simulink model "lin_3d"  (R2020b)
settings: Solver=ode1  StartTime=0.0  StopTime=600  FixedStep=0.001  RelTol=1e-3  EnableMultiTasking=on
values from neighbouring files (symbols this model uses):
  beta3d = 0.9    [simulate_hover.m]
  cycleGain = 0.5    [advanced_model_setup.m]    (also in setup_physical.m = 1; simulate_hover.m = 0.2)
  epsilon3d = evalin('base', 'epsilon3d')    [gainScheduling.m]    (also in simulate_hover.m = 1)
  K = lqi(sys, Q, R)    [gainScheduling.m]    (also in setup_lab_hover.m = K1; simulate_hover.m)
  k3d = evalin('base', 'k3d')    [gainScheduling.m]    (also in simulate_hover.m = 1.65)
  K_AMP = 3    [advanced_model_setup.m]    (also in setup_lab_hover.m; setup_physical.m; simulate_hover.m)
  K_EC_P = 2 * pi / ( 8 * 1024 )    (= 0.000766990393943)    [advanced_model_setup.m]    (also in setup_lab_hover.m; setup_physical.m; simulate_hover.m)
  K_EC_R = 2 * pi / ( 8 * 1024 )    (= 0.000766990393943)    [advanced_model_setup.m]    (also in setup_lab_hover.m; setup_physical.m; simulate_hover.m)
  K_EC_Y = -2 * pi / ( 8 * 1024 )    (= -0.000766990393943)    [advanced_model_setup.m]    (also in setup_lab_hover.m; setup_physical.m; simulate_hover.m)
  u00_range = [-11 -10.5 -10 -9.5 -9 -8.5 -8 -7.5 -7 -6.5 -6 -5.5 ... (45 elements, 1x45)]    [lookup_lin3d.mat]    (also in lookup_nonlin3d.mat; lookup_nonlin_pitchyaw.mat = [-11 -10.9 -10.8 -10.7 -10.6 -10.5 -10.4 -10.3 -10.2 -10.1 -)
  u10_range = -40:0.00001:40    [lookup_gen_5.m]    (also in lookup_gen_optimal.m = -3:0.2:3; lookup_lin3d.mat = [-11 -10.5 -10 -9.5 -9 -8.5 -8 -7.5 -7 -6.5 -6 -5.5 ... (45 ; lookup_nonlin3d.mat = [-11 -10.5 -10 -9.5 -9 -8.5 -8 -7.5 -7 -6.5 -6 -5.5 ... (45 ; lookup_nonlin_pitchyaw.mat = [-11 -10.9 -10.8 -10.7 -10.6 -10.5 -10.4 -10.3 -10.2 -10.1 -)
  u1_T = zeros(x5L, x6L, u10L, u20L)    [lookup_gen_optimal.m]    (also in lookup_lin3d.mat = [-8.91749108301 -9.05775625381 -9.19802070914 -9.33828594207; lookup_nonlin3d.mat = [-10.7844387629 -10.8648620301 -10.9452851893 -11.0257085566; lookup_nonlin_pitchyaw.mat = [-10.9045735396 -10.9207431106 -10.936911981 -10.953081676 -)
  u20_range = -40:0.00001:40    [lookup_gen_5.m]    (also in lookup_gen_optimal.m = -3:0.2:3; lookup_lin3d.mat = [-11 -10.5 -10 -9.5 -9 -8.5 -8 -7.5 -7 -6.5 -6 -5.5 ... (45 ; lookup_nonlin3d.mat = [-11 -10.5 -10 -9.5 -9 -8.5 -8 -7.5 -7 -6.5 -6 -5.5 ... (45 ; lookup_nonlin_pitchyaw.mat = [-11 -10.5 -10 -9.5 -9 -8.5 -8 -7.5 -7 -6.5 -6 -5.5 ... (45 )
  u2_T = zeros(x5L, x6L, u10L, u20L)    [lookup_gen_optimal.m]    (also in lookup_lin3d.mat = [11.9999976349 11.9999976348 11.9999995269 11.9999995269 11.; lookup_nonlin3d.mat = [11.999999986 11.9999999853 11.9999999846 11.9999999837 11.9; lookup_nonlin_pitchyaw.mat = [11.9999999849 11.9999999848 11.9999996928 11.9999999845 11.)
  u3_T = zeros(x5L, x6L, u10L, u20L)    [lookup_gen_optimal.m]    (also in lookup_lin3d.mat = [-11.9999984131 -11.9999984131 -11.9999996826 -11.9999996826; lookup_nonlin3d.mat = [-11.999999986 -11.9999999853 -11.9999999846 -11.9999999837 ; lookup_nonlin_pitchyaw.mat = [-11.9999999699 -11.9999999696 -11.9999993856 -11.999999969 )
  u4_T = zeros(x5L, x6L, u10L, u20L)    [lookup_gen_optimal.m]    (also in lookup_lin3d.mat = [11.9999951772 11.9999951773 11.9999990355 11.9999990356 11.; lookup_nonlin3d.mat = [10.7844387816 10.8648620565 10.9452851985 11.0257085566 11.; lookup_nonlin_pitchyaw.mat = [-11.9999999699 -11.9999999696 -11.9999993856 -11.999999969 )
  V_bias = 12    [advanced_model_setup.m]    (also in setup_lab_hover.m; setup_physical.m; simulate_hover.m)
  VMAX_AMP = 24    [advanced_model_setup.m]    (also in setup_lab_hover.m; setup_physical.m; simulate_hover.m)
  wcf = 2 * pi * 20    (= 125.663706144)    [advanced_model_setup.m]    (also in setup_lab_hover.m; setup_physical.m; simulate_hover.m = 628.318530718)
  x1_traj = x1_traj*pi/180    [lookup_approxLimit.m]    (also in lookup_approxLimit3d.m)
  x1_trajectory = zeros(x1TL, x2TL)    [lookup_approxLimit.m]    (also in lookup_approxLimit3d.m = zeros(x1TL, x2TL, x3TL))
  x2_traj = x2_traj*pi/180    [lookup_approxLimit.m]    (also in lookup_approxLimit3d.m)
  x2_trajectory = zeros(x1TL, x2TL)    [lookup_approxLimit.m]    (also in lookup_approxLimit3d.m = zeros(x1TL, x2TL, x3TL))
  x3_traj = x3_traj*pi/180    [lookup_approxLimit3d.m]
  x3_trajectory = zeros(x1TL, x2TL, x3TL)    [lookup_approxLimit3d.m]
  zetaf = 0.6    [advanced_model_setup.m]    (also in setup_lab_hover.m; setup_physical.m; simulate_hover.m)
undefined symbols (not defined in the file or in its folder): HIL, qc_get_step_size
libraries: simulink_extras x5, quarc_library x3
settings Model: SimulationMode=external  ExtModeTrigDuration=10000  Creator=hpineros  LastModifiedBy=256444
settings SolverCC: PositivePriorityOrder=on
settings DataIOCC: MaxDataPoints=5000  SaveFormat=Array  SignalLoggingSaveFormat=ModelDataLogs  InspectSignalLogs=on  ReturnWorkspaceOutputs=off
settings OptimizationCC: ExpressionDepthLimit=2147483647  InitFltsAndDblsToZero=on  LifeSpan=inf
settings DebuggingCC: SaveWithParameterizedLinksMsg=none  UnderspecifiedInitializationDetection=Classic  MergeDetectMultiDrivingBlocksExec=none  SolverPrmCheckMsg=warning  FcnCallInpInsideContextMsg=warning  StateNameClashWarn=warning  SFUnexpectedBacktrackingDiag=warning  SFNoUnconditionalDefaultTransitionDiag=warning  SFExecutionAtInitializationDiag=none  ArithmeticOperatorsInVariantConditions=warning
settings HardwareCC: ProdBitPerPointer=32  ProdBitPerSizeT=32  ProdBitPerPtrDiffT=32  ProdLargestAtomicFloat=None  ProdIntDivRoundTo=Undefined  ProdEndianess=Unspecified  ProdWordSize=32  ProdHWDeviceType=32-bit Generic
settings ModelReferenceCC: PropagateSignalLabelsOutOfModel=off
settings SFSimCC: SimUseLocalCustomCode=off  CustomCodeUndefinedFunction=UseInterfaceOnly
settings RTWCC: Description=QUARC Win64 Target  SystemTargetFile=quarc_win64.tlc  TemplateMakefile=quarc_default_tmf  RTWUseLocalCustomCode=off
settings CodeAppCC: StateflowObjectComments=on
settings STFCustomTargetCC: CombineOutputUpdateFcns=on  GRTInterface=off
settings GRTTargetCC: TargetLangStandard=C89/C90 (ANSI)  ParMdlRefBuildCompliant=off  CompOptLevelCompliant=off  MatFileLogging=off  UseToolchainInfoCompliant=off  ExtMode=on  ExtModeMexFile=quarc_comm
settings ConfigComp: CovMetricSettings=dw  CovSaveCumulativeToWorkspaceVar=on  CovSaveSingleToWorkspaceVar=on  CovExternalEMLEnable=off

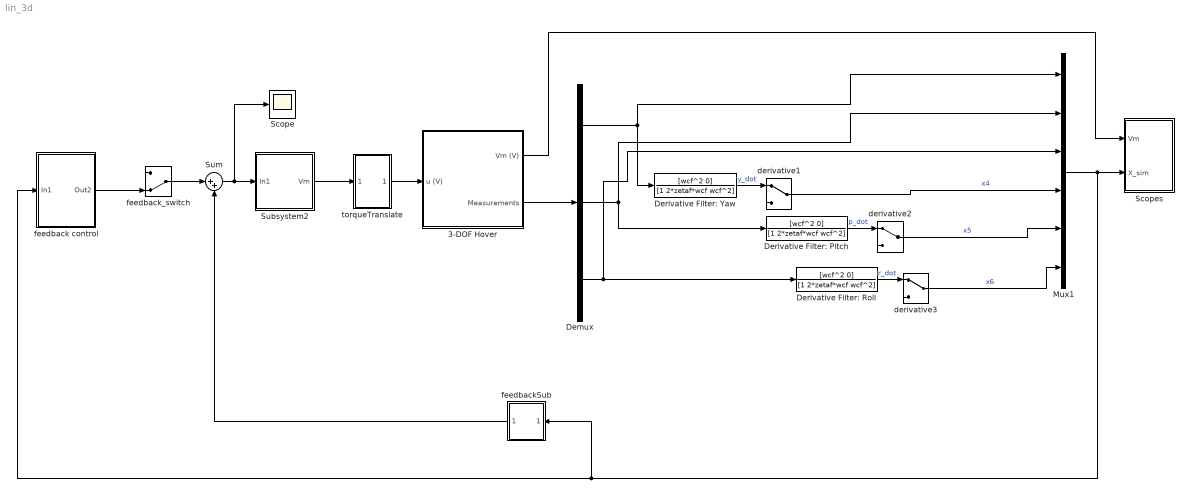
== system lin_3d ==
  3-DOF Hover : Subsystem
  Demux : Demux  Outputs=3
  Derivative Filter: Pitch : TransferFcn  Numerator=[wcf^2 0]  Denominator=[1 2*zetaf*wcf wcf^2]
  Derivative Filter: Roll : TransferFcn  Numerator=[wcf^2 0]  Denominator=[1 2*zetaf*wcf wcf^2]
  Derivative Filter: Yaw : TransferFcn  Numerator=[wcf^2 0]  Denominator=[1 2*zetaf*wcf wcf^2]
  Mux1 : Mux  Inputs=6
  Scope : Scope
  Scopes : Subsystem
  Subsystem2 : Subsystem
  Sum : Sum  Inputs=|++
  derivative1 : ManualSwitch
  derivative2 : ManualSwitch
  derivative3 : ManualSwitch
  feedback control : Subsystem
  feedbackSub : Subsystem
  feedback_switch : ManualSwitch  CurrentSetting=0
  torqueTranslate : Subsystem
  wires:
  Demux/3 -> Mux1/3, Derivative Filter: Roll/1
  Demux/1 -> Mux1/1, Derivative Filter: Yaw/1
  derivative2/1 -> Mux1/5  "x5"
  derivative1/1 -> Mux1/4  "x4"
  Demux/2 -> Mux1/2, Derivative Filter: Pitch/1
  Derivative Filter: Pitch/1 -> derivative2/1  "p_dot"
  Derivative Filter: Roll/1 -> derivative3/1  "r_dot"
  Derivative Filter: Yaw/1 -> derivative1/1  "y_dot"
  3-DOF Hover/2(Measurements) -> Demux/1
  derivative3/1 -> Mux1/6  "x6"
  3-DOF Hover/1(Vm (V)) -> Scopes/1(Vm)
  Mux1/1 -> feedbackSub/1(Input), feedback control/1(In1), Scopes/2(X_sim)
  torqueTranslate/1(Out1) -> 3-DOF Hover/1(u (V))
  feedback_switch/1 -> Sum/1
  feedback control/1(Out2) -> feedback_switch/2
  Sum/1 -> Scope/1, Subsystem2/1(In1)
  Subsystem2/1(Vm) -> torqueTranslate/1(Vm)
  feedbackSub/1(Out1) -> Sum/2

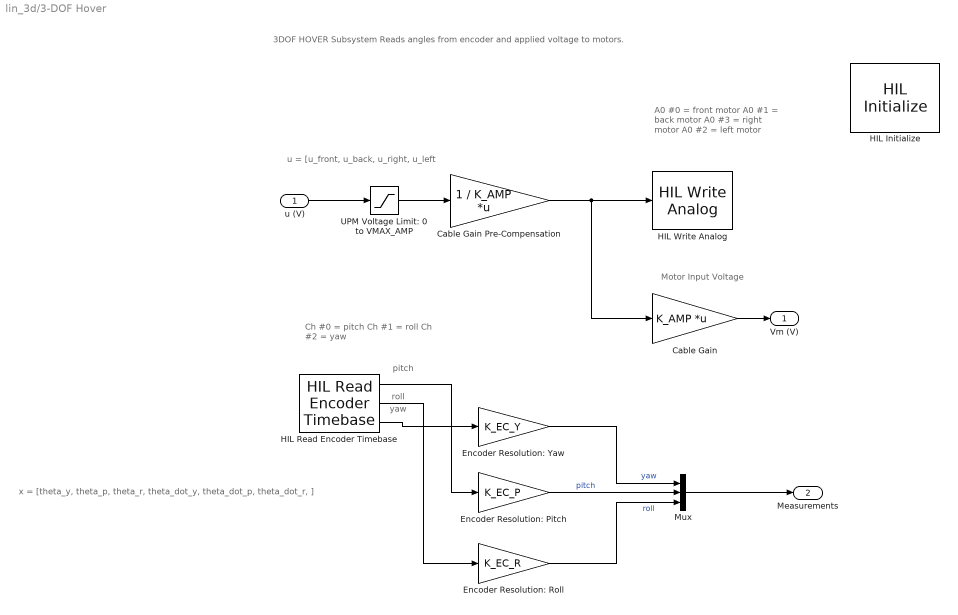
== system lin_3d/3-DOF Hover ==
  note: roll
  note: pitch
  note: yaw
  note: Motor Input Voltage
  note: x = [theta_y, theta_p, theta_r, theta_dot_y, theta_dot_p, theta_dot_r, ]
  note: A0 #0 = front motor
      | A0 #1 = back motor
      | A0 #3 = right motor
      | A0 #2 = left motor
  note: u = [u_front, u_back, u_right, u_left
  note: 3DOF HOVER Subsystem
      | Reads angles from encoder and applied voltage to motors.
  note: Ch #0 = pitch
      | Ch #1 = roll
      | Ch #2 = yaw
  u (V) : Inport
  Cable Gain : Gain  Gain=K_AMP  Multiplication=Matrix(K*u)  SaturateOnIntegerOverflow=on  OutDataTypeStr=Inherit: Same as input  ParamDataTypeStr=Inherit: Same as input
  Cable Gain Pre-Compensation : Gain  Gain=1 / K_AMP  Multiplication=Matrix(K*u)  SaturateOnIntegerOverflow=on  OutDataTypeStr=Inherit: Same as input  ParamDataTypeStr=Inherit: Same as input
  Encoder Resolution: Pitch : Gain  Gain=K_EC_P
  "Encoder Resolution: Roll " : Gain  Gain=K_EC_R
  Encoder Resolution: Yaw : Gain  Gain=K_EC_Y
  HIL Initialize : quarc_library/Data Acquisition/Generic/Configuration/HIL Initialize  object_name=HIL-1  board_type=q8_usb  board_number=0  board_options=update_rate=normal  exclusive=off  active=on  hardware_clocks=[0:2]  clock_modes=[]  initial_clock_frequencies=[]  set_clock_params_at_start=off  set_clock_params_at_switch_in=off  set_clock_frequencies_at_start=off  set_clock_frequencies_at_switch_in=off  analog_input_channels=[0:7]  analog_input_configurations=[]  analog_input_maximums=10  analog_input_minimums=-10  set_analog_input_params_at_start=on  set_analog_input_params_at_switch_in=off  analog_output_channels=[0:7]  analog_output_maximums=10  analog_output_minimums=-10  initial_analog_outputs=[0]  final_analog_outputs=[0]  watchdog_analog_outputs=0  set_analog_output_params_at_start=on  set_analog_output_params_at_switch_in=off  set_analog_outputs_at_start=on  set_analog_outputs_at_switch_in=off  set_analog_outputs_at_terminate=on  set_analog_outputs_at_switch_out=off  set_analog_outputs_on_watchdog=off  digital_input_channels=[]  digital_output_channels=[0:3]  digital_output_configuration=[]  initial_digital_outputs=[0]  final_digital_outputs=[0]  watchdog_digital_outputs=[0]  set_digital_output_params_at_start=off  set_digital_output_params_at_switch_in=off  set_digital_outputs_at_start=on  set_digital_outputs_at_switch_in=off  set_digital_outputs_at_terminate=on  set_digital_outputs_at_switch_out=off  set_digital_outputs_on_watchdog=off  encoder_channels=[0:7]  quadrature=[4]  encoder_filter_frequency=[]  initial_encoder_counts=[0]  set_encoder_params_at_start=on  set_encoder_params_at_switch_in=off  set_encoder_counts_at_start=on  set_encoder_counts_at_switch_in=off  pwm_channels=[0:7]  pwm_modes=0  pwm_frequency=99.532799999999995e6/4095  pwm_configuration=[0]  pwm_alignment=[0]  pwm_polarity=[1]  pwm_leading_deadband=[0]  pwm_trailing_deadband=[0]  initial_pwm_outputs=[0]  final_pwm_outputs=[0]  watchdog_pwm_outputs=[0]  set_pwm_params_at_start=on  set_pwm_params_at_switch_in=off  set_pwm_outputs_at_start=on  set_pwm_outputs_at_switch_in=off  set_pwm_outputs_at_terminate=on  set_pwm_outputs_at_switch_out=off  set_pwm_outputs_on_watchdog=off  other_output_channels=[]  initial_other_outputs=[]  final_other_outputs=[]  watchdog_other_outputs=[]  set_other_outputs_at_start=off  set_other_outputs_at_switch_in=off  set_other_outputs_at_terminate=off  set_other_outputs_at_switch_out=off  set_other_outputs_on_watchdog=off
  HIL Read Encoder Timebase : quarc_library/Data Acquisition/Generic/Timebases/HIL Read Encoder Timebase  object_name=HIL-1  clock=0  channels=[0:2]  active=on  vector_output=off  data_type_mode=Inherit via back propagation  data_type=double  overflow_mode=Error on overflow  samples_in_buffer=max(ceil(1/qc_get_step_size), 1)
  HIL Write Analog : quarc_library/Data Acquisition/Generic/Immediate I//O/HIL Write Analog  object_name=HIL-1  channels=[0,1,2,3]  sample_time=-1  active=off  vector_input=on
  Mux : Mux  Inputs=3
  UPM Voltage Limit: 0 to VMAX_AMP : Saturate  UpperLimit=VMAX_AMP  LowerLimit=0
  Vm (V) : Outport
  Measurements : Outport  Port=2
  wires:
  Cable Gain Pre-Compensation/1 -> Cable Gain/1, HIL Write Analog/1
  HIL Read Encoder Timebase/3 -> Encoder Resolution: Yaw/1
  HIL Read Encoder Timebase/1 -> Encoder Resolution: Pitch/1
  HIL Read Encoder Timebase/2 -> "Encoder Resolution: Roll "/1
  UPM Voltage Limit: 0 to VMAX_AMP/1 -> Cable Gain Pre-Compensation/1
  Cable Gain/1 -> Vm (V)/1
  u (V)/1 -> UPM Voltage Limit: 0 to VMAX_AMP/1
  "Encoder Resolution: Roll "/1 -> Mux/3  "roll"
  Encoder Resolution: Yaw/1 -> Mux/1  "yaw"
  Encoder Resolution: Pitch/1 -> Mux/2  "pitch"
  Mux/1 -> Measurements/1

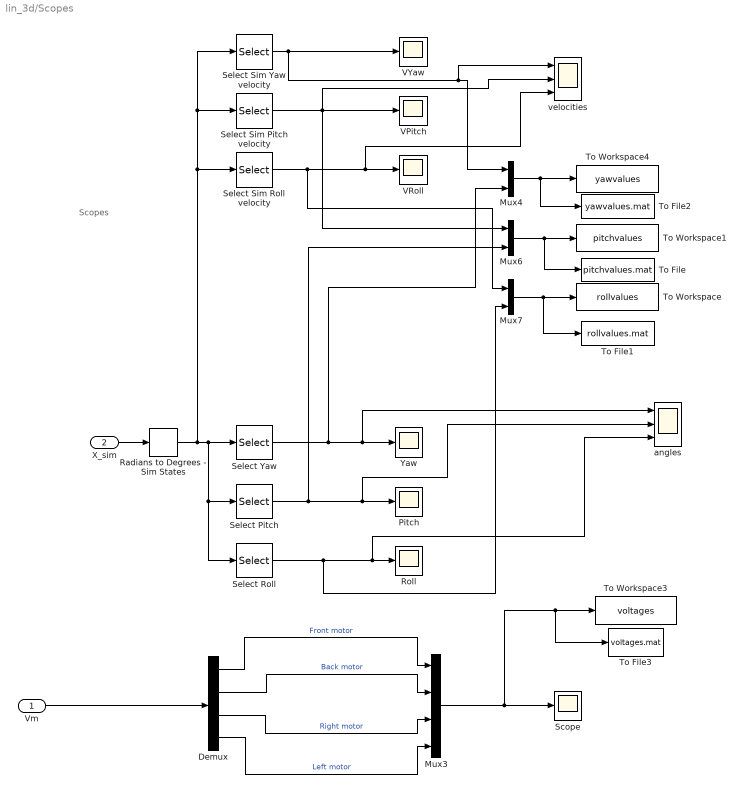
== system lin_3d/Scopes ==
  note: Scopes
  Vm : Inport
  X_sim : Inport  Port=2
  Demux : Demux
  Mux3 : Mux
  Mux4 : Mux  Inputs=2
  Mux6 : Mux  Inputs=2
  Mux7 : Mux  Inputs=2
  Pitch : Scope
  Radians to Degrees - Sim States : simulink_extras/Transformations/Radians to Degrees
  Roll : Scope
  Scope : Scope
  Select Pitch : Selector  InputPortWidth=6  IndexOptions=Index vector (dialog)  Indices=2  OutputSizes=1
  Select Roll : Selector  InputPortWidth=6  IndexOptions=Index vector (dialog)  Indices=3  OutputSizes=1
  Select Sim Pitch velocity : Selector  InputPortWidth=6  IndexOptions=Index vector (dialog)  Indices=5  OutputSizes=1
  Select Sim Roll velocity : Selector  InputPortWidth=6  IndexOptions=Index vector (dialog)  Indices=6  OutputSizes=1
  Select Sim Yaw velocity : Selector  InputPortWidth=6  IndexOptions=Index vector (dialog)  Indices=4  OutputSizes=1
  Select Yaw : Selector  InputPortWidth=6  IndexOptions=Index vector (dialog)  Indices=1  OutputSizes=1
  To File : ToFile  Filename=pitchvalues.mat
  To File1 : ToFile  Filename=rollvalues.mat
  To File2 : ToFile  Filename=yawvalues.mat
  To File3 : ToFile  Filename=voltages.mat
  To Workspace : ToWorkspace  VariableName=rollvalues  SampleTime=-1
  To Workspace1 : ToWorkspace  VariableName=pitchvalues  SampleTime=-1
  To Workspace3 : ToWorkspace  VariableName=voltages  SampleTime=-1
  To Workspace4 : ToWorkspace  VariableName=yawvalues  SampleTime=-1
  VPitch : Scope
  VRoll : Scope
  VYaw : Scope
  Yaw : Scope
  angles : Scope  NumInputPorts=3
  velocities : Scope  NumInputPorts=3
  wires:
  Select Roll/1 -> angles/3, Roll/1, Mux7/2
  Radians to Degrees - Sim States/1 -> Select Sim Roll velocity/1, Select Sim Pitch velocity/1, Select Sim Yaw velocity/1, Select Roll/1, Select Pitch/1, Select Yaw/1
  Select Pitch/1 -> angles/2, Pitch/1, Mux6/2
  X_sim/1 -> Radians to Degrees - Sim States/1
  Demux/1 -> Mux3/1  "Front motor"
  Demux/2 -> Mux3/2  "Back motor"
  Demux/3 -> Mux3/3  "Right motor"
  Demux/4 -> Mux3/4  "Left motor"
  Vm/1 -> Demux/1
  Select Sim Yaw velocity/1 -> VYaw/1, velocities/1, Mux4/1
  Select Sim Roll velocity/1 -> velocities/3, VRoll/1, Mux7/1
  Select Sim Pitch velocity/1 -> Mux6/1, velocities/2, VPitch/1
  Mux3/1 -> To File3/1, To Workspace3/1, Scope/1
  Select Yaw/1 -> angles/1, Yaw/1, Mux4/2
  Mux7/1 -> To File1/1, To Workspace/1
  Mux6/1 -> To File/1, To Workspace1/1
  Mux4/1 -> To File2/1, To Workspace4/1

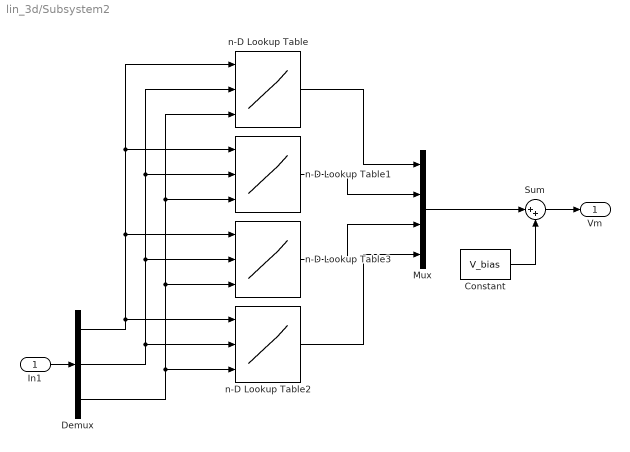
== system lin_3d/Subsystem2 ==
  In1 : Inport
  Constant : Constant  Value=V_bias
  Demux : Demux  Outputs=3
  Mux : Mux
  Sum : Sum  Inputs=|++
  n-D Lookup Table : Lookup_n-D  NumberOfTableDimensions=3  BreakpointsForDimension1=u00_range  BreakpointsForDimension2=u10_range  BreakpointsForDimension3=u20_range  BreakpointsForDimension4=u10_range  BreakpointsForDimension5=u20_range  Table=u1_T  InternalRulePriority=Speed  RndMeth=Simplest  InputSameDT=on
      settings: InputPortMap=u0,u1,u2
  n-D Lookup Table1 : Lookup_n-D  NumberOfTableDimensions=3  BreakpointsForDimension1=u00_range  BreakpointsForDimension2=u10_range  BreakpointsForDimension3=u20_range  BreakpointsForDimension4=u10_range  BreakpointsForDimension5=u20_range  Table=u2_T  InternalRulePriority=Speed  RndMeth=Simplest  InputSameDT=on
      settings: InputPortMap=u0,u1,u2
  n-D Lookup Table2 : Lookup_n-D  NumberOfTableDimensions=3  BreakpointsForDimension1=u00_range  BreakpointsForDimension2=u10_range  BreakpointsForDimension3=u20_range  BreakpointsForDimension4=u10_range  BreakpointsForDimension5=u20_range  Table=u4_T  InternalRulePriority=Speed  RndMeth=Simplest  InputSameDT=on
      settings: InputPortMap=u0,u1,u2
  n-D Lookup Table3 : Lookup_n-D  NumberOfTableDimensions=3  BreakpointsForDimension1=u00_range  BreakpointsForDimension2=u10_range  BreakpointsForDimension3=u20_range  BreakpointsForDimension4=u10_range  BreakpointsForDimension5=u20_range  Table=u3_T  InternalRulePriority=Speed  RndMeth=Simplest  InputSameDT=on
      settings: InputPortMap=u0,u1,u2
  Vm : Outport
  wires:
  Sum/1 -> Vm/1
  Mux/1 -> Sum/1
  Constant/1 -> Sum/2
  In1/1 -> Demux/1
  n-D Lookup Table/1 -> Mux/1
  n-D Lookup Table1/1 -> Mux/2
  n-D Lookup Table3/1 -> Mux/3
  n-D Lookup Table2/1 -> Mux/4
  Demux/1 -> n-D Lookup Table2/1, n-D Lookup Table3/1, n-D Lookup Table/1, n-D Lookup Table1/1
  Demux/3 -> n-D Lookup Table2/3, n-D Lookup Table3/3, n-D Lookup Table1/3, n-D Lookup Table/3
  Demux/2 -> n-D Lookup Table2/2, n-D Lookup Table3/2, n-D Lookup Table1/2, n-D Lookup Table/2

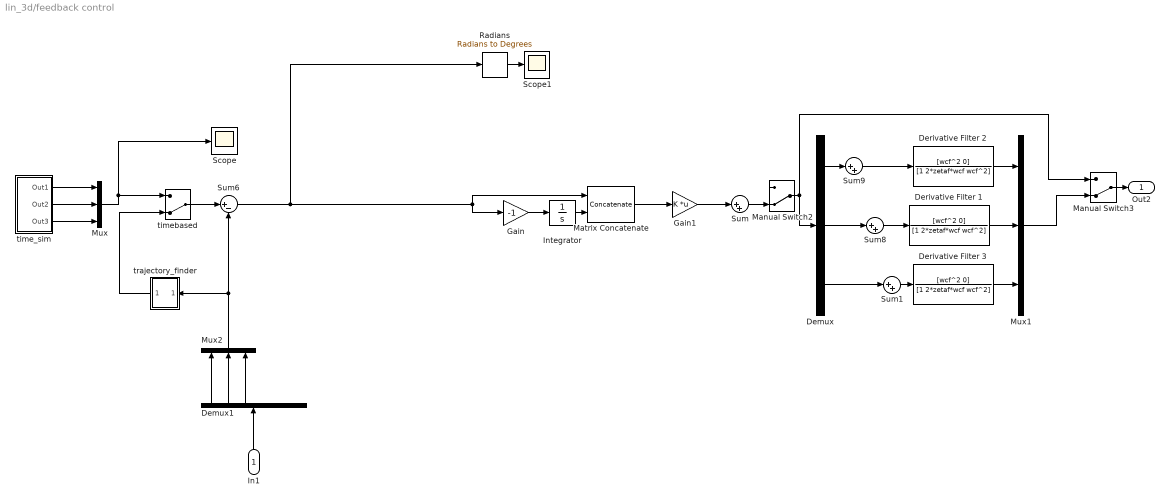
== system lin_3d/feedback control ==
  In1 : Inport
  Demux : Demux  Outputs=3
  Demux1 : Demux  Outputs=6
  Derivative Filter 1 : TransferFcn  Numerator=[wcf^2 0]  Denominator=[1 2*zetaf*wcf wcf^2]
  Derivative Filter 2 : TransferFcn  Numerator=[wcf^2 0]  Denominator=[1 2*zetaf*wcf wcf^2]
  Derivative Filter 3 : TransferFcn  Numerator=[wcf^2 0]  Denominator=[1 2*zetaf*wcf wcf^2]
  Gain : Gain  Gain=-1
  Gain1 : Gain  Gain=K  Multiplication=Matrix(K*u)
  Integrator : Integrator
  Manual Switch2 : ManualSwitch  CurrentSetting=0
  Manual Switch3 : ManualSwitch  CurrentSetting=0
  Matrix Concatenate : Concatenate  Mode=Multidimensional array
  Mux : Mux  Inputs=3
  Mux1 : Mux  Inputs=3
  Mux2 : Mux  Inputs=3
  Radians : simulink_extras/Transformations/Radians to Degrees
  Scope : Scope
  Scope1 : Scope
  Sum{,1,8..9} (4 alike) : Sum  Inputs=|++
  Sum6 : Sum  Inputs=|+-
  time_sim : Subsystem
  timebased : ManualSwitch  CurrentSetting=0
  trajectory_finder : Subsystem
  Out2 : Outport
  wires:
  Mux/1 -> timebased/1, Scope/1
  Demux1/2 -> Mux2/2
  Demux1/1 -> Mux2/1
  Demux1/3 -> Mux2/3
  In1/1 -> Demux1/1
  Mux2/1 -> Sum6/2, trajectory_finder/1(Input)
  time_sim/1(Out1) -> Mux/1
  time_sim/2(Out2) -> Mux/2
  time_sim/3(Out3) -> Mux/3
  Demux/1 -> Sum9/1
  Demux/2 -> Sum8/1
  Derivative Filter 1/1 -> Mux1/2
  Manual Switch3/1 -> Out2/1
  Radians/1 -> Scope1/1
  Sum/1 -> Manual Switch2/2
  Manual Switch2/1 -> Manual Switch3/1, Demux/1
  Derivative Filter 2/1 -> Mux1/1
  Sum8/1 -> Derivative Filter 1/1
  Mux1/1 -> Manual Switch3/2
  Sum9/1 -> Derivative Filter 2/1
  Sum1/1 -> Derivative Filter 3/1
  Derivative Filter 3/1 -> Mux1/3
  Demux/3 -> Sum1/1
  timebased/1 -> Sum6/1
  trajectory_finder/1(Output) -> timebased/2
  Sum6/1 -> Radians/1, Matrix Concatenate/1, Gain/1
  Gain/1 -> Integrator/1
  Integrator/1 -> Matrix Concatenate/2
  Gain1/1 -> Sum/1
  Matrix Concatenate/1 -> Gain1/1

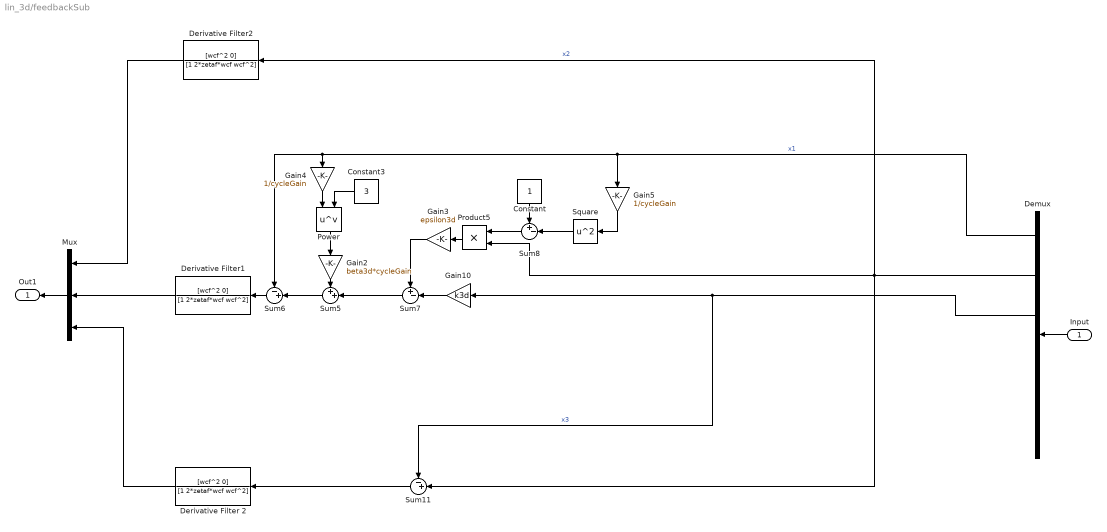
== system lin_3d/feedbackSub ==
  Input : Inport
  Constant : Constant
  Constant3 : Constant  Value=3
  Demux : Demux  Outputs=6
  Derivative Filter 2 : TransferFcn  Numerator=[wcf^2 0]  Denominator=[1 2*zetaf*wcf wcf^2]
  Derivative Filter1 : TransferFcn  Numerator=[wcf^2 0]  Denominator=[1 2*zetaf*wcf wcf^2]
  Derivative Filter2 : TransferFcn  Numerator=[wcf^2 0]  Denominator=[1 2*zetaf*wcf wcf^2]
  Gain10 : Gain  Gain=k3d
  Gain2 : Gain  Gain=beta3d*cycleGain
  Gain3 : Gain  Gain=epsilon3d
  Gain4 : Gain  Gain=1/cycleGain
  Gain5 : Gain  Gain=1/cycleGain
  Mux : Mux  Inputs=3
  Power : Math  Operator=pow  SaturateOnIntegerOverflow=on
  Product5 : Product
  Square : Math  Operator=square  SaturateOnIntegerOverflow=on
  Sum11 : Sum  Inputs=-+|
  Sum5 : Sum  Inputs=++|
  Sum6 : Sum  Inputs=-+|
  Sum7 : Sum  Inputs=+-|
  Sum8 : Sum  Inputs=+-|
  Out1 : Outport
  wires:
  Input/1 -> Demux/1
  Sum7/1 -> Sum5/2
  Sum5/1 -> Sum6/2
  Gain4/1 -> Power/1
  Demux/1 -> Sum6/1, Gain4/1, Gain5/1  "x1"
  Gain5/1 -> Square/1
  Product5/1 -> Gain3/1
  Sum6/1 -> Derivative Filter1/1
  Power/1 -> Gain2/1
  Constant3/1 -> Power/2
  Gain10/1 -> Sum7/2
  Constant/1 -> Sum8/1
  Sum8/1 -> Product5/1
  Square/1 -> Sum8/2
  Gain2/1 -> Sum5/1
  Gain3/1 -> Sum7/1
  Sum11/1 -> Derivative Filter 2/1
  Demux/3 -> Sum11/1, Gain10/1  "x3"
  Demux/2 -> Derivative Filter2/1, Product5/2, Sum11/2  "x2"
  Derivative Filter2/1 -> Mux/1
  Derivative Filter1/1 -> Mux/2
  Derivative Filter 2/1 -> Mux/3
  Mux/1 -> Out1/1

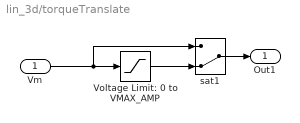
== system lin_3d/torqueTranslate ==
  Vm : Inport
  Voltage Limit: 0 to VMAX_AMP : Saturate  UpperLimit=VMAX_AMP  LowerLimit=0
  sat1 : ManualSwitch  CurrentSetting=0
  Out1 : Outport
  wires:
  Voltage Limit: 0 to VMAX_AMP/1 -> sat1/2
  sat1/1 -> Out1/1
  Vm/1 -> sat1/1, Voltage Limit: 0 to VMAX_AMP/1

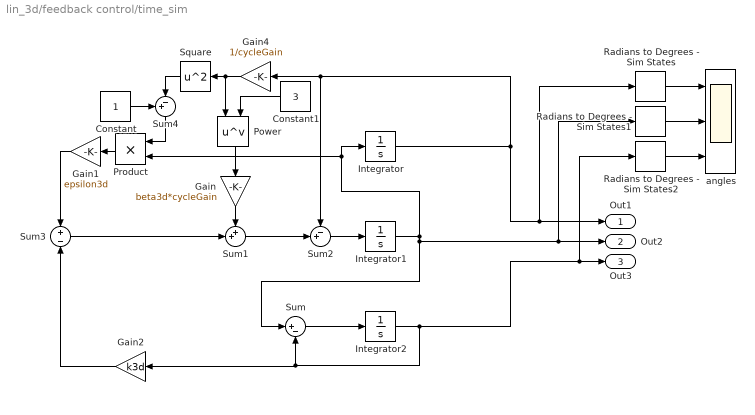
== system lin_3d/feedback control/time_sim ==
  Constant : Constant
  Constant1 : Constant  Value=3
  Gain : Gain  Gain=beta3d*cycleGain
  Gain1 : Gain  Gain=epsilon3d
  Gain2 : Gain  Gain=k3d
  Gain4 : Gain  Gain=1/cycleGain
  Integrator : Integrator  InitialCondition=0.0001
  Integrator1 : Integrator  InitialCondition=0.0001
  Integrator2 : Integrator  InitialCondition=0.0001
  Power : Math  Operator=pow  SaturateOnIntegerOverflow=on
  Product : Product
  Radians to Degrees - Sim States : simulink_extras/Transformations/Radians to Degrees
  Radians to Degrees - Sim States1 : simulink_extras/Transformations/Radians to Degrees
  Radians to Degrees - Sim States2 : simulink_extras/Transformations/Radians to Degrees
  Square : Math  Operator=square  SaturateOnIntegerOverflow=on
  Sum : Sum  Inputs=|+-
  Sum1 : Sum  Inputs=++|
  Sum2 : Sum  Inputs=-+|
  Sum3 : Sum  Inputs=+|-
  Sum4 : Sum  Inputs=+-|
  angles : Scope  NumInputPorts=3
  Out1 : Outport
  Out2 : Outport  Port=2
  Out3 : Outport  Port=3
  wires:
  Gain4/1 -> Square/1, Power/1
  Product/1 -> Gain1/1
  Constant/1 -> Sum4/1
  Sum3/1 -> Sum1/2
  Sum2/1 -> Integrator1/1
  Gain/1 -> Sum1/1
  Gain2/1 -> Sum3/2
  Square/1 -> Sum4/2
  Sum1/1 -> Sum2/2
  Power/1 -> Gain/1
  Gain1/1 -> Sum3/1
  Constant1/1 -> Power/2
  Sum/1 -> Integrator2/1
  Integrator2/1 -> Radians to Degrees - Sim States2/1, Out3/1, Sum/2, Gain2/1
  Sum4/1 -> Product/1
  Integrator1/1 -> Radians to Degrees - Sim States1/1, Out2/1, Sum/1, Product/2, Integrator/1
  Integrator/1 -> Out1/1, Radians to Degrees - Sim States/1, Gain4/1, Sum2/1
  Radians to Degrees - Sim States/1 -> angles/1
  Radians to Degrees - Sim States1/1 -> angles/2
  Radians to Degrees - Sim States2/1 -> angles/3

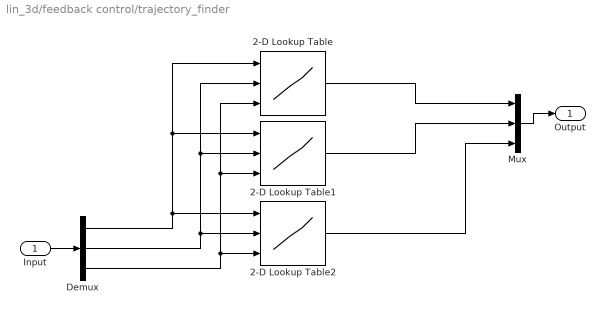
== system lin_3d/feedback control/trajectory_finder ==
  Input : Inport
  2-D Lookup Table : Lookup_n-D  NumberOfTableDimensions=3  BreakpointsForDimension1=x1_traj  BreakpointsForDimension2=x2_traj  BreakpointsForDimension3=x3_traj  Table=x1_trajectory  InternalRulePriority=Speed  RndMeth=Simplest  InputSameDT=on
      settings: InputPortMap=u0,u1,u2
  2-D Lookup Table1 : Lookup_n-D  NumberOfTableDimensions=3  BreakpointsForDimension1=x1_traj  BreakpointsForDimension2=x2_traj  BreakpointsForDimension3=x3_traj  Table=x2_trajectory  InternalRulePriority=Speed  RndMeth=Simplest  InputSameDT=on
      settings: InputPortMap=u0,u1,u2
  2-D Lookup Table2 : Lookup_n-D  NumberOfTableDimensions=3  BreakpointsForDimension1=x1_traj  BreakpointsForDimension2=x2_traj  BreakpointsForDimension3=x3_traj  Table=x3_trajectory  InternalRulePriority=Speed  RndMeth=Simplest  InputSameDT=on
      settings: InputPortMap=u0,u1,u2
  Demux : Demux  Outputs=3
  Mux : Mux  Inputs=3
  Output : Outport
  wires:
  2-D Lookup Table/1 -> Mux/1
  Demux/1 -> 2-D Lookup Table2/1, 2-D Lookup Table/1, 2-D Lookup Table1/1
  2-D Lookup Table1/1 -> Mux/2
  Mux/1 -> Output/1
  Input/1 -> Demux/1
  2-D Lookup Table2/1 -> Mux/3
  Demux/2 -> 2-D Lookup Table/2, 2-D Lookup Table1/2, 2-D Lookup Table2/2
  Demux/3 -> 2-D Lookup Table/3, 2-D Lookup Table1/3, 2-D Lookup Table2/3
